simulink model "full_triped_test"  (R2021a)
settings: Solver=daessc  StartTime=0.0  StopTime=300  RelTol=1e-3
undefined symbols (not defined in the file or in its folder): X, Y, Z
libraries: nesl_utility x10, sm_lib x9, spsFirstOrderFilterLib x4, TripedLibrary x4
settings Model: Creator=jan-b  LastModifiedBy=jan-b
settings SolverCC: AlgebraicLoopSolver=TrustRegion
settings DebuggingCC: SFMachineParentedDataDiag=warning

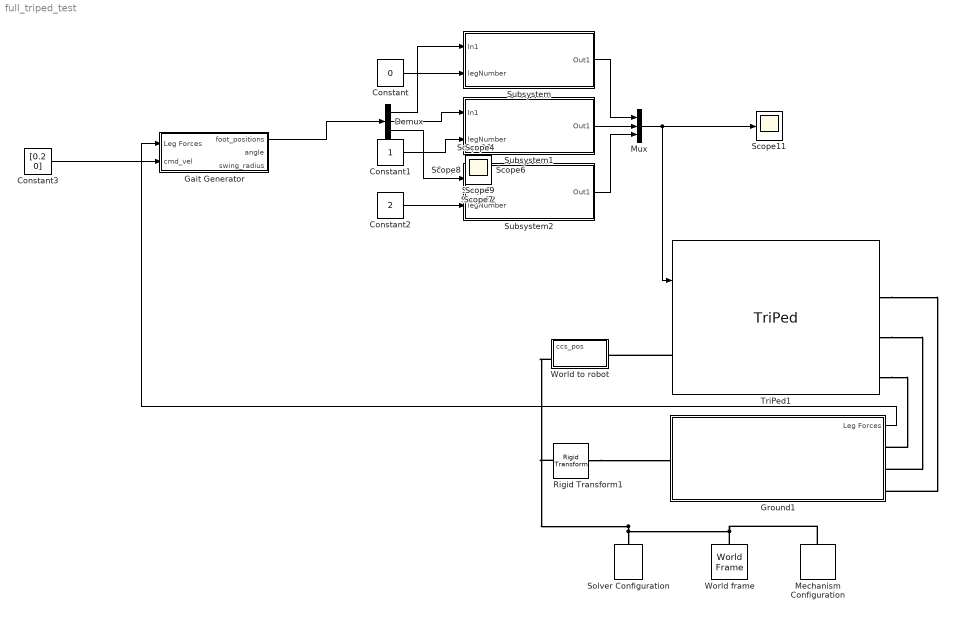
== system full_triped_test ==
  Constant : Constant  Value=0
  Constant1 : Constant
  Constant2 : Constant  Value=2
  Constant3 : Constant  Value=[0.2 0]
  Demux : Demux  Outputs=3
  Gait Generator : Subsystem
  Ground1 : Subsystem
  Mechanism Configuration : sm_lib/Utilities/Mechanism Configuration  UniformGravity=Constant  GravityVector=[0 0 -9.80665]  GravityVectorUnits=m/s^2  GravityUnits=m/s^2  LinearizationDelta=0.001  JointModeTransitionNonlinearIterations=2
  Mux : Mux  Inputs=3
  Rigid Transform1 : sm_lib/Frames and Transforms/Rigid Transform  TranslationMethod=Cartesian  TranslationStandardOffset=-0.7  TranslationLengthUnit=m  TranslationStandardAxis=+Z  TranslationCartesianOffset="[1.5  0 -0.7]"  TranslationROffset=0  TranslationROffsetUnits=m  TranslationZOffset=0  TranslationZOffsetUnits=m  TranslationThetaOffset=0  TranslationThetaOffsetUnits=deg  RotationMethod=None  RotationAngleUnits=deg  RotationStandardAxis=+Z  RotationAngle=0.0  RotationArbitraryAxis=[0 0 1]  FollAlignAxisA=+X  BaseAlignAxisA=+Y  FollAlignAxisB=+Y  BaseAlignAxisB=+Z  RotationSequenceAxes=FollowerAxes  RotationSequence=XYX  RotationSequenceAngles=[0 0 0]  RotationSequenceAnglesUnits=deg  RotationMatrix=[1 0 0; 0 1 0; 0 0 1]
  Scope{,1..12} (13 alike) : Scope
  Solver Configuration : nesl_utility/Solver Configuration  PhysicalDomain=network_engine_domain  SubClassName=solver  LeftPortType=input  RightPortType=generic  Tones=[]  Harmonics=[]  SimulateNoise=off  Profile=off  UseLocalSampling=off  EnableSwitchedLinearOptims=on  FrequencyDomain=off  UseCCode=off  RelTol=0.001  AbsTol=1e-06  MinStep=1e-09  ToWorkspace=off  RevertToSquareIcSolve=off  NumHomotopyIterations=100  PhasorMode=off  PhasorModeNumHarmonics=1  DoDC=off  ResidualTolerance=1e-09  UseLocalSolver=off  LocalSolverChoice=NE_BACKWARD_EULER_ADVANCER  LocalSolverSampleTime=0.001  DoFixedCost=off  MaxNonlinIter=3  MaxModeIter=2  ComputeImpulses=off  ImpulseIterations=2  LinearAlgebra=Sparse  EquationFormulation=NE_TIME_EF  DelaysMemoryBudget=1024  AutomaticFiltering=on  FilteringTimeConstant=0.001  PartitionStorageMethod=AS_NEEDED  PartitionMemoryBudget=1024  PartitionMethod=FAST
      settings: SourceProductBaseCode=PW,SS
  Subsystem : Subsystem
  Subsystem1 : Subsystem
  Subsystem2 : Subsystem
  TriPed1 : TripedLibrary/Full Model/TriPed  SystemSampleTime=-1  VariantActivationTime=update diagram  Latency=0  AutoFrameSizeCalculation=off
      settings: SourceProductName=TriPed Library
  World frame : sm_lib/Frames and Transforms/World Frame
  World to robot : Subsystem  VariantControl=Choice_2
      settings: PortSchema="{\"entries\":[{\"content\":{\"sides\":[{\"content\":{\"connectorIds\":[\"Out1\",\"LConn1\"]},\"type\":\"ConnectorPlacement.EquallySpacedRectSide\",\"uuid\":\"fa97ec4b-bb52-439b-9a14-1527e54f4313\"},{\"content\":{\"connectorIds\":[\"RConn1\"],\"side\":\"RIGHT\"},\"type\":\"ConnectorPlacement.EquallySpacedRectSide\",\"uuid\":\"748595cb-ce69-4b14-8a7b-6533d5cde02d\"},{\"content\":{\"connectorIds\":[],\"side\":\"TOP\"},\"type\":\"ConnectorPlacement.EquallySpacedRectSide\",\"uuid\":\"beff1859-f326-4ae5-8410-6df9adae8922\"}]},\"type\":\"ConnectorPlacement.EquallySpacedConnector\",\"uuid\":\"2d140454-e8b6-4875-b494-9efb77071119\"}],\"packageUris\":[\"http://schema.mathworks.com/mf0/Connector/R2020b\"],\"version\":\"1.0\"}"
  wires:
  Gait Generator/1(foot_positions) -> Demux/1
  Ground1/1(Leg Forces) -> Gait Generator/1(Leg Forces)
  Demux/1 -> Subsystem/1(In1)
  Demux/2 -> Subsystem1/1(In1)
  Demux/3 -> Subsystem2/1(In1)
  Constant/1 -> Subsystem/2(legNumber)
  Constant1/1 -> Subsystem1/2(legNumber)
  Constant2/1 -> Subsystem2/2(legNumber)
  Subsystem/1(Out1) -> Mux/1
  Subsystem1/1(Out1) -> Mux/2
  Subsystem2/1(Out1) -> Mux/3
  Mux/1 -> Scope11/1, TriPed1/1
  Constant3/1 -> Gait Generator/2(cmd_vel)
  connections:
  Solver Configuration/RConn1 -- World to robot/LConn1 -- Rigid Transform1/LConn1 -- Mechanism Configuration/RConn1 -- World frame/RConn1
  Rigid Transform1/RConn1 -- Ground1/LConn1
  TriPed1/LConn1 -- World to robot/RConn1
  TriPed1/RConn1 -- Ground1/RConn3
  TriPed1/RConn2 -- Ground1/RConn2
  TriPed1/RConn3 -- Ground1/RConn1

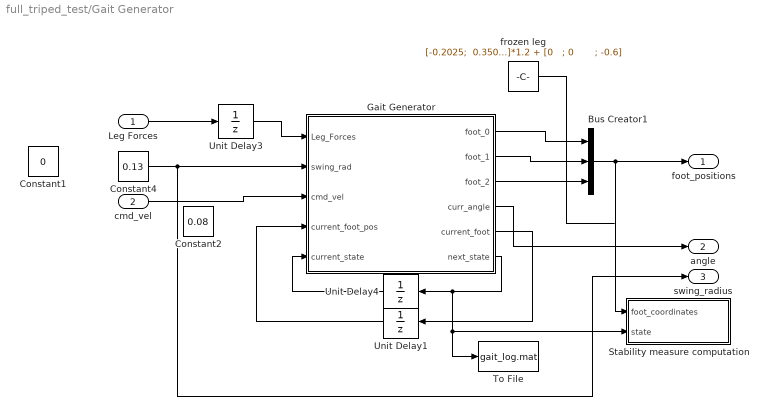
== system full_triped_test/Gait Generator ==
  Leg Forces : Inport
  cmd_vel : Inport  Port=2
  Bus Creator1 : BusCreator  Inputs=3
  Constant1 : Constant  Value=0
  Constant2 : Constant  Value=0.08
  Constant4 : Constant  Value=0.13
  Gait Generator : MATLAB Function  TreatAsAtomicUnit=on  SystemSampleTime=0.01
  Stability measure computation : Subsystem
  To File : ToFile  Filename=gait_log.mat  MatrixName=gait_log  SaveFormat=Timeseries
  Unit Delay1 : UnitDelay  InitialCondition=[0 0 0 0 0 0 0 0 0 0 0 0]  SampleTime=-1  HasFrameUpgradeWarning=on
  Unit Delay3 : UnitDelay  InitialCondition=[0 0 0]  SampleTime=-1  HasFrameUpgradeWarning=on
  Unit Delay4 : UnitDelay  InitialCondition=[2 2 2]  SampleTime=-1  HasFrameUpgradeWarning=on
  frozen leg : Constant  Value="[-0.2025;  0.35074;  -0]*1.2 + [0   ; 0       ; -0.6]"
  foot_positions : Outport
  angle : Outport  Port=2
  swing_radius : Outport  Port=3
  wires:
  Bus Creator1/1 -> Stability measure computation/1(foot_coordinates), foot_positions/1
  Gait Generator/1(foot_0) -> Bus Creator1/1
  Gait Generator/2(foot_1) -> Bus Creator1/2
  Gait Generator/3(foot_2) -> Bus Creator1/3
  Unit Delay1/1 -> Gait Generator/4(current_foot_pos)
  Gait Generator/4(curr_angle) -> angle/1
  cmd_vel/1 -> Gait Generator/3(cmd_vel)
  Gait Generator/5(current_foot) -> Unit Delay1/1
  Constant4/1 -> Gait Generator/2(swing_rad), swing_radius/1
  Leg Forces/1 -> Unit Delay3/1
  Unit Delay3/1 -> Gait Generator/1(Leg_Forces)
  Gait Generator/6(next_state) -> To File/1, Stability measure computation/2(state), Unit Delay4/1
  Unit Delay4/1 -> Gait Generator/5(current_state)
  frozen leg/1 -> ?

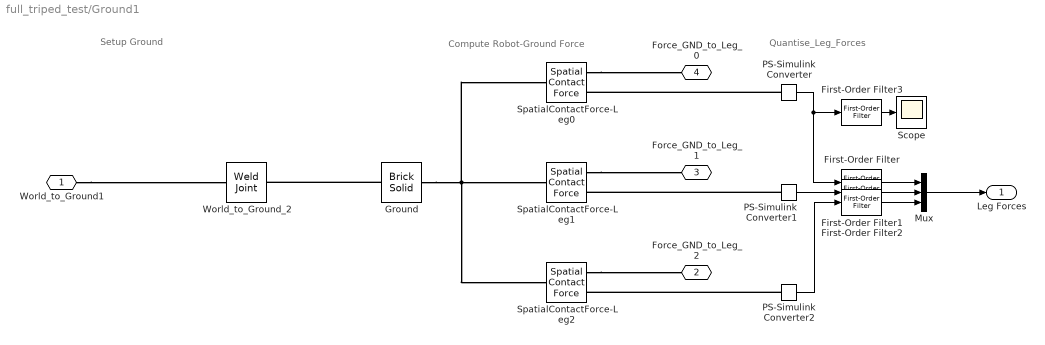
== system full_triped_test/Ground1 ==
  note: Setup Ground
  note: Compute Robot-Ground Force
  note: Quantise_Leg_Forces
  First-Order Filter : spsFirstOrderFilterLib/First-Order Filter  FilterType=Lowpass  Tc=1/30  Ts=0  Initialize=on  Vac_Init=[0, 0, 60]  Vdc_Init=0  PlotResponse=off  FreqRange="[0,  200,  1]"
  First-Order Filter1 : spsFirstOrderFilterLib/First-Order Filter  FilterType=Lowpass  Tc=1/30  Ts=0  Initialize=on  Vac_Init=[0, 0, 60]  Vdc_Init=0  PlotResponse=off  FreqRange="[0,  200,  1]"
  First-Order Filter2 : spsFirstOrderFilterLib/First-Order Filter  FilterType=Lowpass  Tc=1/30  Ts=0  Initialize=on  Vac_Init=[0, 0, 60]  Vdc_Init=0  PlotResponse=off  FreqRange="[0,  200,  1]"
  First-Order Filter3 : spsFirstOrderFilterLib/First-Order Filter  FilterType=Lowpass  Tc=1/5  Ts=0  Initialize=on  Vac_Init=[0, 0, 60]  Vdc_Init=0  PlotResponse=off  FreqRange="[0,  200,  1]"
  Ground : sm_lib/Body Elements/Brick Solid  GraphicAmbientColor=[0.15 0.15 0.15 1.0]  BasedOnType=Density  BrickDimensions=[5 5 0.1]  BrickDimensionUnits=m  CenterOfMass=[0 0 0]  CenterOfMassUnits=m  GraphicDiffuseColor=[0.4 0.4 0.4]  Density=1000  DensityUnits=kg/m^3  DoExposeReferenceFrame=on  GraphicEmissiveColor=[0.0 0.0 0.0 1.0]  ExportEntireGeometry=on  SerializedFrames=<Frames/>  MarkerShape=Sphere  MarkerSize=10  GraphicType=FromGeometry  InertiaType=CalculateFromGeometry  Mass=1  MassUnits=kg  MomentsOfInertia=[1 1 1]  MomentsOfInertiaUnits=kg*m^2  GraphicOpacity=0.8  ProductsOfInertia=[0 0 0]  ProductsOfInertiaUnits=kg*m^2  GraphicShininess=75  GraphicSpecularColor=[0.5 0.5 0.5 1.0]  GraphicVisPropType=SimpleVisualProperties
  Mux : Mux  Inputs=3
  PS-Simulink Converter : nesl_utility/PS-Simulink Converter  PhysicalDomain=network_engine_domain  SubClassName=ps_output  LeftPortType=input  RightPortType=output  PseudoPeriodic=off  Frequencies=[]  Unit=inherit  AffineConversion=off
      settings: SourceProductBaseCode=PW,SS
  PS-Simulink Converter1 : nesl_utility/PS-Simulink Converter  PhysicalDomain=network_engine_domain  SubClassName=ps_output  LeftPortType=input  RightPortType=output  PseudoPeriodic=off  Frequencies=[]  Unit=inherit  AffineConversion=off
      settings: SourceProductBaseCode=PW,SS
  PS-Simulink Converter2 : nesl_utility/PS-Simulink Converter  PhysicalDomain=network_engine_domain  SubClassName=ps_output  LeftPortType=input  RightPortType=output  PseudoPeriodic=off  Frequencies=[]  Unit=inherit  AffineConversion=off
      settings: SourceProductBaseCode=PW,SS
  Scope : Scope
  SpatialContactForce-Leg0 : sm_lib/Forces and Torques/Spatial Contact Force  CoefficientOfDynamicFriction=0.6  CoefficientOfStaticFriction=1  SenseContactBaseRotation=off  SenseContactBaseTranslation=off  NormalDamping=10^3  NormalDampingUnits=N/(m/s)  SenseContactFollowerRotation=off  SenseContactFollowerTranslation=off  SenseContactSignal=off  NormalStiffness=30000  NormalStiffnessUnits=N/m  FrictionalCriticalVelocity=1e-2  FrictionalCriticalVelocityUnits=m/s  ZeroCrossDetectContactStartAndEnd=on  FrictionType=SmoothStickSlip  SenseFrictionalForceMagnitude=off  SenseNormalForceMagnitude=on  NormalForceType=SmoothSpringDamper  SenseNormalVelocity=off  SenseSeparationDistance=off  SenseTangentialVelocity=off  SenseTangentialVelocityMagnitude=off  NormalTransitionRegionWidth=1e-3  NormalTransitionRegionWidthUnits=m
  SpatialContactForce-Leg1 : sm_lib/Forces and Torques/Spatial Contact Force  CoefficientOfDynamicFriction=0.6  CoefficientOfStaticFriction=1  SenseContactBaseRotation=off  SenseContactBaseTranslation=off  NormalDamping=10^3  NormalDampingUnits=N/(m/s)  SenseContactFollowerRotation=off  SenseContactFollowerTranslation=off  SenseContactSignal=off  NormalStiffness=30000  NormalStiffnessUnits=N/m  FrictionalCriticalVelocity=1e-2  FrictionalCriticalVelocityUnits=m/s  ZeroCrossDetectContactStartAndEnd=on  FrictionType=SmoothStickSlip  SenseFrictionalForceMagnitude=off  SenseNormalForceMagnitude=on  NormalForceType=SmoothSpringDamper  SenseNormalVelocity=off  SenseSeparationDistance=off  SenseTangentialVelocity=off  SenseTangentialVelocityMagnitude=off  NormalTransitionRegionWidth=1e-3  NormalTransitionRegionWidthUnits=m
  SpatialContactForce-Leg2 : sm_lib/Forces and Torques/Spatial Contact Force  CoefficientOfDynamicFriction=0.6  CoefficientOfStaticFriction=1  SenseContactBaseRotation=off  SenseContactBaseTranslation=off  NormalDamping=10^3  NormalDampingUnits=N/(m/s)  SenseContactFollowerRotation=off  SenseContactFollowerTranslation=off  SenseContactSignal=off  NormalStiffness=30000  NormalStiffnessUnits=N/m  FrictionalCriticalVelocity=1e-2  FrictionalCriticalVelocityUnits=m/s  ZeroCrossDetectContactStartAndEnd=on  FrictionType=SmoothStickSlip  SenseFrictionalForceMagnitude=off  SenseNormalForceMagnitude=on  NormalForceType=SmoothSpringDamper  SenseNormalVelocity=off  SenseSeparationDistance=off  SenseTangentialVelocity=off  SenseTangentialVelocityMagnitude=off  NormalTransitionRegionWidth=1e-3  NormalTransitionRegionWidthUnits=m
  World_to_Ground_2 : sm_lib/Joints/Weld Joint  JointMode=Normal  SenseConstraintForce=off  SenseConstraintForceX=off  SenseConstraintForceY=off  SenseConstraintForceZ=off  SenseConstraintTorque=off  SenseConstraintTorqueX=off  SenseConstraintTorqueY=off  SenseConstraintTorqueZ=off  SenseTotalForce=off  SenseTotalForceX=off  SenseTotalForceY=off  SenseTotalForceZ=off  SenseTotalTorque=off  SenseTotalTorqueX=off  SenseTotalTorqueY=off  SenseTotalTorqueZ=off  CompositeWrenchDir=FollowerOnBase  CompositeWrenchFrame=BaseFrame
  World_to_Ground1 : PMIOPort  Side=Left
  Force_GND_to_Leg_2 : PMIOPort  Port=2  Side=Right
  Force_GND_to_Leg_1 : PMIOPort  Port=3  Side=Right
  Force_GND_to_Leg_0 : PMIOPort  Port=4  Side=Right
  Leg Forces : Outport
  wires:
  PS-Simulink Converter/1 -> First-Order Filter3/1, First-Order Filter/1
  PS-Simulink Converter1/1 -> First-Order Filter1/1
  PS-Simulink Converter2/1 -> First-Order Filter2/1
  Mux/1 -> Leg Forces/1
  First-Order Filter/1 -> Mux/1
  First-Order Filter1/1 -> Mux/2
  First-Order Filter2/1 -> Mux/3
  First-Order Filter3/1 -> Scope/1
  connections:
  Ground/RConn1 -- World_to_Ground_2/RConn1
  Ground/LConn1 -- SpatialContactForce-Leg0/LConn1 -- SpatialContactForce-Leg1/LConn1 -- SpatialContactForce-Leg2/LConn1
  SpatialContactForce-Leg1/RConn1 -- Force_GND_to_Leg_1/RConn1
  SpatialContactForce-Leg2/RConn1 -- Force_GND_to_Leg_2/RConn1
  SpatialContactForce-Leg0/RConn1 -- Force_GND_to_Leg_0/RConn1
  World_to_Ground1/RConn1 -- World_to_Ground_2/LConn1
  PS-Simulink Converter1/LConn1 -- SpatialContactForce-Leg1/RConn2
  PS-Simulink Converter2/LConn1 -- SpatialContactForce-Leg2/RConn2
  PS-Simulink Converter/LConn1 -- SpatialContactForce-Leg0/RConn2

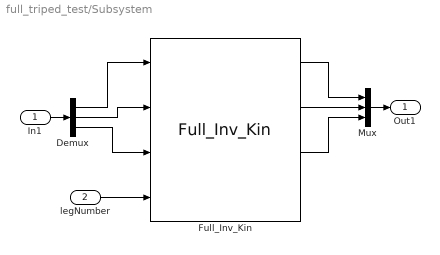
== system full_triped_test/Subsystem ==
  In1 : Inport
  legNumber : Inport  Port=2
  Demux : Demux  Outputs=3
  Full_Inv_Kin : TripedLibrary/Kinematic Utils/Full Model kinematics/Full_Inv_Kin  SystemSampleTime=-1  VariantActivationTime=update diagram  Latency=0  AutoFrameSizeCalculation=off
      settings: SourceProductName=TriPed Library
  Mux : Mux  Inputs=3
  Out1 : Outport
  wires:
  Demux/1 -> Full_Inv_Kin/1
  Full_Inv_Kin/3 -> Mux/3
  Full_Inv_Kin/1 -> Mux/1
  Demux/2 -> Full_Inv_Kin/2
  Demux/3 -> Full_Inv_Kin/3
  In1/1 -> Demux/1
  Full_Inv_Kin/2 -> Mux/2
  Mux/1 -> Out1/1
  legNumber/1 -> Full_Inv_Kin/4

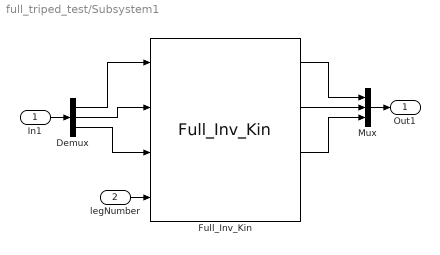
== system full_triped_test/Subsystem1 ==
  In1 : Inport
  legNumber : Inport  Port=2
  Demux : Demux  Outputs=3
  Full_Inv_Kin : TripedLibrary/Kinematic Utils/Full Model kinematics/Full_Inv_Kin  SystemSampleTime=-1  VariantActivationTime=update diagram  Latency=0  AutoFrameSizeCalculation=off
      settings: SourceProductName=TriPed Library
  Mux : Mux  Inputs=3
  Out1 : Outport
  wires:
  Demux/1 -> Full_Inv_Kin/1
  Full_Inv_Kin/3 -> Mux/3
  Full_Inv_Kin/1 -> Mux/1
  Demux/2 -> Full_Inv_Kin/2
  Demux/3 -> Full_Inv_Kin/3
  In1/1 -> Demux/1
  Full_Inv_Kin/2 -> Mux/2
  Mux/1 -> Out1/1
  legNumber/1 -> Full_Inv_Kin/4

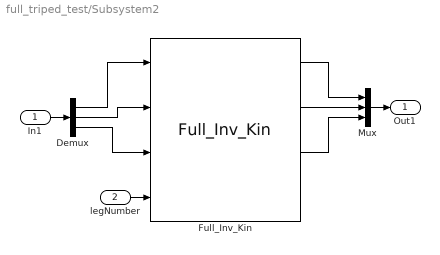
== system full_triped_test/Subsystem2 ==
  In1 : Inport
  legNumber : Inport  Port=2
  Demux : Demux  Outputs=3
  Full_Inv_Kin : TripedLibrary/Kinematic Utils/Full Model kinematics/Full_Inv_Kin  SystemSampleTime=-1  VariantActivationTime=update diagram  Latency=0  AutoFrameSizeCalculation=off
      settings: SourceProductName=TriPed Library
  Mux : Mux  Inputs=3
  Out1 : Outport
  wires:
  Demux/1 -> Full_Inv_Kin/1
  Full_Inv_Kin/3 -> Mux/3
  Full_Inv_Kin/1 -> Mux/1
  Demux/2 -> Full_Inv_Kin/2
  Demux/3 -> Full_Inv_Kin/3
  In1/1 -> Demux/1
  Full_Inv_Kin/2 -> Mux/2
  Mux/1 -> Out1/1
  legNumber/1 -> Full_Inv_Kin/4

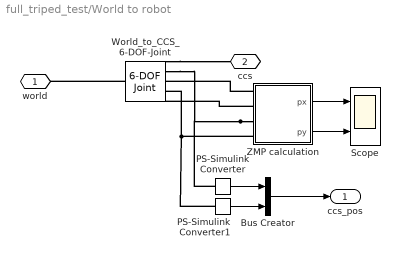
== system full_triped_test/World to robot ==
  Bus Creator : BusCreator  Inputs=2
  PS-Simulink Converter : nesl_utility/PS-Simulink Converter  PhysicalDomain=network_engine_domain  SubClassName=ps_output  LeftPortType=input  RightPortType=output  PseudoPeriodic=off  Frequencies=[]  Unit=inherit  AffineConversion=off
      settings: SourceProductBaseCode=PW,SS
  PS-Simulink Converter1 : nesl_utility/PS-Simulink Converter  PhysicalDomain=network_engine_domain  SubClassName=ps_output  LeftPortType=input  RightPortType=output  PseudoPeriodic=off  Frequencies=[]  Unit=inherit  AffineConversion=off
      settings: SourceProductBaseCode=PW,SS
  Scope : Scope  NumInputPorts=2
  World_to_CCS_6-DOF-Joint : sm_lib/Joints/6-DOF Joint  JointMode=Normal  SenseConstraintForce=off  SenseConstraintForceX=off  SenseConstraintForceY=off  SenseConstraintForceZ=off  SenseConstraintTorque=off  SenseConstraintTorqueX=off  SenseConstraintTorqueY=off  SenseConstraintTorqueZ=off  SenseTotalForce=off  SenseTotalForceX=off  SenseTotalForceY=off  SenseTotalForceZ=off  SenseTotalTorque=off  SenseTotalTorqueX=off  SenseTotalTorqueY=off  SenseTotalTorqueZ=off  CompositeWrenchDir=FollowerOnBase  CompositeWrenchFrame=BaseFrame  PxEquilibriumPosition=0  PxEquilibriumPositionUnits=m  PxSpringStiffness=0  PxSpringStiffnessUnits=N/m  PxDampingCoefficient=0  PxDampingCoefficientUnits=N/(m/s)  PxTorqueActuationMode=NoTorque  PxMotionActuationMode=ComputedMotion  PxSensePosition=on  PxSenseVelocity=off  PxSenseAcceleration=on  PxSenseTorqueForce=off  PxSenseLowerLimitTorqueForce=off  PxSenseUpperLimitTorqueForce=off  PxLowerLimitSpecify=off  PxLowerLimitBound=-1  PxLowerLimitBoundUnits=m  PxLowerLimitStiffness=1e6  PxLowerLimitStiffnessUnits=N/m  PxLowerLimitDamping=1e3  PxLowerLimitDampingUnits=N/(m/s)  PxLowerLimitTransitionRegionWidth=1e-4  PxLowerLimitTransitionRegionWidthUnits=m  PxUpperLimitSpecify=off  PxUpperLimitBound=1  PxUpperLimitBoundUnits=m  PxUpperLimitStiffness=1e6  PxUpperLimitStiffnessUnits=N/m  PxUpperLimitDamping=1e3  PxUpperLimitDampingUnits=N/(m/s)  PxUpperLimitTransitionRegionWidth=1e-4  PxUpperLimitTransitionRegionWidthUnits=m  PxPositionTargetSpecify=off  PxPositionTargetPriority=High  PxPositionTargetValue=0  PxPositionTargetValueUnits=m  PxVelocityTargetSpecify=off  PxVelocityTargetPriority=High  PxVelocityTargetValue=0  PxVelocityTargetValueUnits=m/s  PyEquilibriumPosition=0  PyEquilibriumPositionUnits=m  PySpringStiffness=0  PySpringStiffnessUnits=N/m  PyDampingCoefficient=0  PyDampingCoefficientUnits=N/(m/s)  PyTorqueActuationMode=NoTorque  PyMotionActuationMode=ComputedMotion  PySensePosition=on  PySenseVelocity=off  PySenseAcceleration=on  PySenseTorqueForce=off  PySenseLowerLimitTorqueForce=off  PySenseUpperLimitTorqueForce=off  PyLowerLimitSpecify=off  PyLowerLimitBound=-1  PyLowerLimitBoundUnits=m  PyLowerLimitStiffness=1e6  PyLowerLimitStiffnessUnits=N/m  PyLowerLimitDamping=1e3  PyLowerLimitDampingUnits=N/(m/s)  PyLowerLimitTransitionRegionWidth=1e-4  PyLowerLimitTransitionRegionWidthUnits=m  PyUpperLimitSpecify=off  PyUpperLimitBound=1  PyUpperLimitBoundUnits=m  PyUpperLimitStiffness=1e6  PyUpperLimitStiffnessUnits=N/m  PyUpperLimitDamping=1e3  PyUpperLimitDampingUnits=N/(m/s)  PyUpperLimitTransitionRegionWidth=1e-4  PyUpperLimitTransitionRegionWidthUnits=m  PyPositionTargetSpecify=off  PyPositionTargetPriority=High  PyPositionTargetValue=0  PyPositionTargetValueUnits=m  PyVelocityTargetSpecify=off  PyVelocityTargetPriority=High  PyVelocityTargetValue=0  PyVelocityTargetValueUnits=m/s  PzEquilibriumPosition=0  PzEquilibriumPositionUnits=m  PzSpringStiffness=0  PzSpringStiffnessUnits=N/m  PzDampingCoefficient=0  PzDampingCoefficientUnits=N/(m/s)  PzTorqueActuationMode=NoTorque  PzMotionActuationMode=ComputedMotion  PzSensePosition=off  PzSenseVelocity=off  PzSenseAcceleration=off  PzSenseTorqueForce=off  PzSenseLowerLimitTorqueForce=off  PzSenseUpperLimitTorqueForce=off  PzLowerLimitSpecify=off  PzLowerLimitBound=-1  PzLowerLimitBoundUnits=m  PzLowerLimitStiffness=1e6  PzLowerLimitStiffnessUnits=N/m  PzLowerLimitDamping=1e3  PzLowerLimitDampingUnits=N/(m/s)  PzLowerLimitTransitionRegionWidth=1e-4  PzLowerLimitTransitionRegionWidthUnits=m  PzUpperLimitSpecify=off  PzUpperLimitBound=1  PzUpperLimitBoundUnits=m  PzUpperLimitStiffness=1e6  PzUpperLimitStiffnessUnits=N/m  PzUpperLimitDamping=1e3  PzUpperLimitDampingUnits=N/(m/s)  PzUpperLimitTransitionRegionWidth=1e-4  PzUpperLimitTransitionRegionWidthUnits=m  PzPositionTargetSpecify=off  PzPositionTargetPriority=High  PzPositionTargetValue=0  PzPositionTargetValueUnits=m  PzVelocityTargetSpecify=off  PzVelocityTargetPriority=High  PzVelocityTargetValue=0  PzVelocityTargetValueUnits=m/s  SphDefPosRotationMethod=None  SphDefPosRotationAngleUnits=deg  SphDefPosRotationStandardAxis=+Z  SphDefPosRotationAngle=0.0  SphDefPosRotationArbitraryAxis=[0 0 1]  SphDefPosFollAlignAxisA=+X  SphDefPosBaseAlignAxisA=+Y  SphDefPosFollAlignAxisB=+Y  SphDefPosBaseAlignAxisB=+Z  SphDefPosRotationSequenceAxes=FollowerAxes  SphDefPosRotationSequence=XYX  SphDefPosRotationSequenceAngles=[0 0 0]  SphDefPosRotationSequenceAnglesUnits=deg  SphDefPosRotationMatrix=[1 0 0; 0 1 0; 0 0 1]  SphEqPosRotationMethod=None  SphEqPosRotationAngleUnits=deg  SphEqPosRotationStandardAxis=+Z  SphEqPosRotationAngle=0.0  SphEqPosRotationArbitraryAxis=[0 0 1]  SphEqPosFollAlignAxisA=+X  SphEqPosBaseAlignAxisA=+Y  SphEqPosFollAlignAxisB=+Y  SphEqPosBaseAlignAxisB=+Z  SphEqPosRotationSequenceAxes=FollowerAxes  SphEqPosRotationSequence=XYX  SphEqPosRotationSequenceAngles=[0 0 0]  SphEqPosRotationSequenceAnglesUnits=deg  SphEqPosRotationMatrix=[1 0 0; 0 1 0; 0 0 1]  SphSpringStiffness=0  SphSpringStiffnessUnits=N*m/deg  SphDampingCoefficient=0  SphDampingCoefficientUnits=N*m/(deg/s)  SphActuateTorqueX=off  SphActuateTorqueY=off  SphActuateTorqueZ=off  SphActuateTorque=off  SphTorqueActuationMode=NoTorque  SphMotionActuationMode=ComputedMotion  SphActuationFrame=BaseFrame  SphSensePosition=off  SphSenseVelocityX=off  SphSenseVelocityY=off  SphSenseVelocityZ=off  SphSenseVelocity=off  SphSenseAccelerationX=off  SphSenseAccelerationY=off  SphSenseAccelerationZ=off  SphSenseAcceleration=off  SphSenseTorqueX=off  SphSenseTorqueY=off  SphSenseTorqueZ=off  SphSenseTorqueForce=off  SphSenseLowerLimitTorqueMag=off  SphSenseUpperLimitTorqueMag=off  SphSensingFrame=BaseFrame  SphLowerLimitSpecify=off  SphLowerLimitBound=15  SphLowerLimitBoundUnits=deg  SphLowerLimitStiffness=1e4  SphLowerLimitStiffnessUnits=N*m/deg  SphLowerLimitDamping=10  SphLowerLimitDampingUnits=N*m/(deg/s)  SphLowerLimitTransitionRegionWidth=0.1  SphLowerLimitTransitionRegionWidthUnits=deg  SphUpperLimitSpecify=off  SphUpperLimitBound=45  SphUpperLimitBoundUnits=deg  SphUpperLimitStiffness=1e4  SphUpperLimitStiffnessUnits=N*m/deg  SphUpperLimitDamping=10  SphUpperLimitDampingUnits=N*m/(deg/s)  SphUpperLimitTransitionRegionWidth=0.1  SphUpperLimitTransitionRegionWidthUnits=deg  SphPositionTargetRotationMethod=None  SphPositionTargetRotationAngleUnits=deg  SphPositionTargetRotationStandardAxis=+Z  SphPositionTargetRotationAngle=0.0  SphPositionTargetRotationArbitraryAxis=[0 0 1]  SphPositionTargetFollAlignAxisA=+X  SphPositionTargetBaseAlignAxisA=+Y  SphPositionTargetFollAlignAxisB=+Y  SphPositionTargetBaseAlignAxisB=+Z  SphPositionTargetRotationSequenceAxes=FollowerAxes  SphPositionTargetRotationSequence=XYX  SphPositionTargetRotationSequenceAngles=[0 0 0]  SphPositionTargetRotationSequenceAnglesUnits=deg  SphPositionTargetRotationMatrix=[1 0 0; 0 1 0; 0 0 1]  SphPositionTargetSpecify=off  SphPositionTargetPriority=High  SphVelocityTargetValue=[0 0 0]  SphVelocityTargetValueUnits=deg/s  SphVelocityTargetSpecify=off  SphVelocityTargetPriority=High  SphVelocityTargetInFollowerFrame=on
  ZMP calculation : Subsystem
  world : PMIOPort  Side=Left
  ccs : PMIOPort  Port=2  Side=Right
  ccs_pos : Outport
  wires:
  ZMP calculation/1(px) -> Scope/1
  ZMP calculation/2(py) -> Scope/2
  Bus Creator/1 -> ccs_pos/1
  PS-Simulink Converter/1 -> Bus Creator/1
  PS-Simulink Converter1/1 -> Bus Creator/2
  connections:
  World_to_CCS_6-DOF-Joint/RConn1 -- ccs/RConn1
  World_to_CCS_6-DOF-Joint/LConn1 -- world/RConn1
  ZMP calculation/LConn3 -- World_to_CCS_6-DOF-Joint/RConn2 -- PS-Simulink Converter/LConn1
  ZMP calculation/LConn1 -- World_to_CCS_6-DOF-Joint/RConn3
  ZMP calculation/LConn4 -- World_to_CCS_6-DOF-Joint/RConn4 -- PS-Simulink Converter1/LConn1
  ZMP calculation/LConn2 -- World_to_CCS_6-DOF-Joint/RConn5

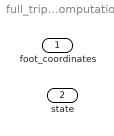
== system full_triped_test/Gait Generator/Stability measure computation ==
  foot_coordinates : Inport
  state : Inport  Port=2

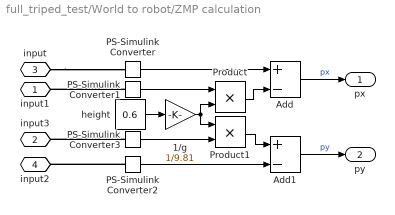
== system full_triped_test/World to robot/ZMP calculation ==
  1/g : Gain  Gain=1/9.81
  Add : Sum  Inputs=+-
  Add1 : Sum  Inputs=+-
  PS-Simulink Converter{,1..3} (4 alike) : nesl_utility/PS-Simulink Converter  PhysicalDomain=network_engine_domain  SubClassName=ps_output  LeftPortType=input  RightPortType=output  PseudoPeriodic=off  Frequencies=[]  Unit=inherit  AffineConversion=off
      settings: SourceProductBaseCode=PW,SS
  Product : Product
  Product1 : Product
  height : Constant  Value=0.6
  input1 : PMIOPort  Side=Left
  input3 : PMIOPort  Port=2  Side=Left
  input : PMIOPort  Port=3  Side=Left
  input2 : PMIOPort  Port=4  Side=Left
  px : Outport
  py : Outport  Port=2
  wires:
  height/1 -> 1/g/1
  PS-Simulink Converter1/1 -> Product/1
  1/g/1 -> Product1/1, Product/2
  PS-Simulink Converter3/1 -> Product1/2
  Product/1 -> Add/2
  Product1/1 -> Add1/1
  PS-Simulink Converter2/1 -> Add1/2
  PS-Simulink Converter/1 -> Add/1
  Add1/1 -> py/1  "py"
  Add/1 -> px/1  "px"
  connections:
  input/RConn1 -- PS-Simulink Converter/LConn1
  PS-Simulink Converter2/LConn1 -- input2/RConn1
  PS-Simulink Converter3/LConn1 -- input3/RConn1
  PS-Simulink Converter1/LConn1 -- input1/RConn1

== matlab function full_triped_test/Gait Generator/Gait Generator ==
  data: Leg_Forces input; swing_rad input; cmd_vel input; foot_0 output; foot_1 output; foot_2 output; curr_angle output; current_foot_pos input; current_foot output; next_state output; current_state input
function [foot_0,foot_1,foot_2,curr_angle,current_foot, next_state] = fcn(Leg_Forces, swing_rad,cmd_vel,current_foot_pos, current_state)


    initial_pos_0 = [0.4    ; 0       ;  -0]*1.2 + [0   ; 0       ; -0.6];
    initial_pos_1 = [-0.2025; -0.35074;  -0]*1.2 + [0   ; 0       ; -0.6];
    initial_pos_2 = [-0.2025;  0.35074;  -0]*1.2 + [0   ; 0       ; -0.6];
    

    
    current_foot= [0;0;0;0;0;0;0;0;0;0;0;0];
    next_state=current_state;

    
    persistent angle
    if isempty(angle)
        angle = [-2*pi;-2*pi;-2*pi];
    end
    curr_angle =angle(1);
    
    persistent last_step_angle
    if isempty(last_step_angle)
        last_step_angle = [0;0;0];
    end
 
    persistent last_step_vel
    if isempty(last_step_vel)
        last_step_vel = [0;0;0;0;0;0];
    end

    persistent step_pos
    if isempty(step_pos)
        step_pos = [initial_pos_0;initial_pos_1;initial_pos_2];
    end
    
    
   [foot_0,current_foot(1:4) ,next_state(1),last_step_angle(1),last_step_vel(1:2),step_pos(1:3),angle(1)]  = single_leg_state_machine(initial_pos_0,last_step_vel(1:2),last_step_angle(1),current_state(1),current_foot_pos(1:4) ,step_pos(1:3),angle(1),swing_rad,cmd_vel,Leg_Forces,1);
   [foot_1,current_foot(5:8) ,next_state(2),last_step_angle(2),last_step_vel(3:4),step_pos(4:6),angle(2)]  = single_leg_state_machine(initial_pos_1,last_step_vel(3:4),last_step_angle(2),current_state(2),current_foot_pos(5:8) ,step_pos(4:6),angle(2),swing_rad,cmd_vel,Leg_Forces,2);  
   [foot_2,current_foot(9:12),next_state(3),last_step_angle(3),last_step_vel(5:6),step_pos(7:9),angle(3)]  = single_leg_state_machine(initial_pos_2,last_step_vel(5:6),last_step_angle(3),current_state(3),current_foot_pos(9:12),step_pos(7:9),angle(3),swing_rad,cmd_vel,Leg_Forces,3);


end

function [foot,current_liftoff,next_state,current_step,last_vel,step_pos,angle]=single_leg_state_machine(initial_pos,last_vel,prev_step,current_state,foot_pos,step_pos,last_angle,swing_rad,cmd_vel,all_forces,leg_numb)

timestep    = 0.01;
increment   = 2;%1.75;%pi;
angle       = last_angle+increment*timestep;

height= 0.05;
step_time= 1.2;%1;
timestep  = 0.01;


[rad_walking_dir,velocity]=cart2pol(cmd_vel(1),cmd_vel(2));
walking_dir=rad_walking_dir/(2*pi)*360;
velocity = velocity/increment;

rel_step_angle=step_time/increment/timestep;
    

corrected_foot   = foot_pos(1:3)-swing_rad*[cos(angle);sin(angle);0]; %foot in ECCS

move_memory=angle-prev_step;


switch (current_state)
    case 0
        init_angle    = foot_pos(4);
        final_angle   = init_angle+2*pi/360*rel_step_angle;
        s = angdiff(angle,init_angle)/angdiff(final_angle,init_angle);
       
        
        if (s<=1)
            next_state = 0;
            current_step = prev_step+2.5*0.01;
        else
            next_state =1;
            current_step = angle;

        end
        
        est_trvl=max((2*pi-move_memory)/increment,0);
        final_pos    = initial_pos+swing_rad*[cos(final_angle);sin(final_angle);0] + rotz(last_vel(2))*[1;0;0]*est_trvl*last_vel(1)/2;
        foot         = targeted_step(s,height,foot_pos(1:3),final_pos);
        current_liftoff = foot_pos; 
        step_pos  = initial_pos + rotz(last_vel(2))*[1;0;0]*est_trvl*last_vel(1)/2;

        
    case 1
        %mapping circuit inputs onto [-1,1] (a type of fuzzyfication)
        force         = all_forces(leg_numb);
        %low_force     = 1-1/(1+exp(-0.5*(force-40)));
        force = 1/(1+exp(-0.05*(force-15)));

        low_force     = 1-force;
        actuator_ampl = 1/(1+exp(-90*(move_memory*velocity-0.04)));
        
        if INVOKE(actuator_ampl,low_force) >= 0.92%%0.94%0.99%0.994   
            next_state =0;
        else
            next_state = 1;
        end
        foot = step_pos+swing_rad*[cos(angle);sin(angle);0]-rotz(walking_dir)*[1;0;0]*move_memory*velocity; %TODO should be full roll pitch yaw control
        current_liftoff = [foot;angle];
        current_step = prev_step;
        last_vel = [velocity;walking_dir];
        
    % initialisation case to allow the simulation to settle
    case 2
        if angle >= 0
            next_state=1;
        else
            next_state=2;    
        end
        foot = initial_pos+(2*pi+angle)/(2*pi)*swing_rad*[cos(0);sin(0);0];
        current_liftoff = [foot;0]; 
        current_step = prev_step;
        
    otherwise
         next_state      = current_state;
         
         foot            = foot_pos(1:3);
         current_liftoff = foot_pos; 
         current_step = prev_step;
end
end


function foot_position=targeted_step(s,height,start,stop)
    relative_pos  = stop-start;
    [rot,len]   = cart2pol(relative_pos(1),relative_pos(2));
    foot_position = rotz(rot/(2*pi)*360)*step(s,len,height)+start;
end

function foot_position=step(s,length,height)

z  = height*exp(-(s-0.5)^2/0.01);%0.01
%z   = height*(-(s-0.5)^2+0.25)*4;
%z   = height*(1/(1+exp(-40*(s+0.4-0.5)))-1/(1+exp(-20*(s-0.1-0.5))));
%x = 0.5* length*(1+(sign(s-0.5)*sqrt(1-z^2/height^2)));
x = length/(1+exp(-20*(s-0.5)));
y = 0; 

foot_position = [x; y; z];
end


function activation = OR(x,y)
d=1;
activation=tanh(d*(x+y))/tanh(d*2); 
end

function activation = AND(x,y)
d=1;
activation = tanh(d*(x+y-OR(x,y)))/tanh(d*1);
end

function activation = INVOKE(x,y)
activation = AND(x,OR(x,y));
end

function activation  = PREVAIL(x,y)
activation = OR(x,OR(x,y));
end

function activation = COMPARE(x,y)
activation = OR(x,-y);
end

function activation=XOR(x,y)
activation = 2*COMPARE(x,y).^2.*OR(x,y);
end
